simulink model "ButterWorth_filter"  (R2017a)
settings: Solver=FixedStepAuto  StartTime=0.0  StopTime=duracao  FixedStep=0.008  RelTol=1e-3
undefined symbols (not defined in the file or in its folder): a, b
settings Model: Creator=pedro  LastModifiedBy=pedro

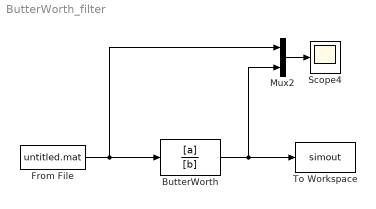
== system ButterWorth_filter ==
  "ButterWorth " : TransferFcn  Numerator=[a]  Denominator=[b]
  From File : FromFile  SampleTime=0
  Mux2 : Mux  Inputs=2
  Scope4 : Scope
  To Workspace : ToWorkspace  VariableName=simout  SampleTime=-1
  wires:
  From File/1 -> Mux2/1, "ButterWorth "/1
  "ButterWorth "/1 -> Mux2/2, To Workspace/1
  Mux2/1 -> Scope4/1
